simulink model "SKKP"  (R2014b)
settings: Solver=ode113  StartTime=0.0  StopTime=400  FixedStep=0.1  RelTol=1e-1  AbsTol=1e-1
undefined symbols (not defined in the file or in its folder): deg, eps_max, eps_min, H3dm, H4dm, Jdm, L, M3dm, M4dm, Newton, P, R0, rad, Raphson, s, Td, Tpp, V0, y_out
libraries: aerolibconvert2 x26, aerolibtransform2 x19, aerolibutil x7, aerolibobsolete x6, dspinverses x5, vrlib x1, aerolib6dof2 x1
(part 2 of 2)

== system SKKP/Фильтр калмана w  ==
  wizm : Inport
  wtek : Inport  Port=2
  Angular Velocity Conversion1 : aerolibconvert2/Angular Velocity Conversion  IU=rad/s  OU=deg/s
  Demux1 : Demux  Outputs=3
  Demux2 : Demux  Outputs=3
  MATLAB Function : MATLAB Function  TreatAsAtomicUnit=on
  MATLAB Function1 : MATLAB Function  TreatAsAtomicUnit=on
  MATLAB Function2 : MATLAB Function  TreatAsAtomicUnit=on
  Mux : Mux  Inputs=3
  wfilt : Outport
  wires:
  Demux1/1 -> MATLAB Function/2(meas)
  MATLAB Function1/2(yhatOut) -> Mux/2
  MATLAB Function/2(yhatOut) -> Mux/1
  MATLAB Function2/2(yhatOut) -> Mux/3
  Demux2/3 -> MATLAB Function2/1(u)
  Demux2/2 -> MATLAB Function1/1(u)
  Demux1/2 -> MATLAB Function1/2(meas)
  Demux2/1 -> MATLAB Function/1(u)
  Mux/1 -> Angular Velocity Conversion1/1
  wtek/1 -> Demux2/1
  Demux1/3 -> MATLAB Function2/2(meas)
  wizm/1 -> Demux1/1
  Angular Velocity Conversion1/1 -> wfilt/1

== system SKKP/АД/Перевод из углов в кватернионы1 ==
  fi : Inport
  Angle Conversion1 : aerolibconvert2/Angle Conversion  IU=deg  OU=rad
  Rotation Angles to Quaternions1 : aerolibtransform2/Rotation Angles to Quaternions  rotationOrder=ZYX
  Selector1 : Selector  InputPortWidth=3  Indices=[3 2 1]
  q : Outport
  wires:
  Angle Conversion1/1 -> Rotation Angles to Quaternions1/1
  Selector1/1 -> Angle Conversion1/1
  Rotation Angles to Quaternions1/1 -> q/1
  fi/1 -> Selector1/1

== system SKKP/ГИВУС/Subsystem ==
  ЧЭ1 : Inport
  ЧЭ2 : Inport  Port=2
  ЧЭ3 : Inport  Port=3
  ЧЭ4 : Inport  Port=4
  Gain4 : Gain
  wпск : Outport
  wires:
  Gain4/1 -> wпск/1
  ЧЭ1/1 -> Gain4/1

== system SKKP/Задание моментов инерции/Разворот 1 ==
  j : Inport
  Action Port : ActionPort  ActionType=then
  "j  " : Outport
  wires:
  j/1 -> "j  "/1

== system SKKP/Задание моментов инерции/Разворот 10 ==
  "j " : Inport
  Action Port : ActionPort  ActionType=then
  "j  " : Outport
  wires:
  "j "/1 -> "j  "/1

== system SKKP/Задание моментов инерции/Разворот 2 ==
  j : Inport
  Action Port : ActionPort  ActionType=then
  "j  " : Outport
  wires:
  j/1 -> "j  "/1

== system SKKP/Задание моментов инерции/Разворот 3 ==
  j : Inport
  Action Port : ActionPort  ActionType=then
  "j  " : Outport
  wires:
  j/1 -> "j  "/1

== system SKKP/Задание моментов инерции/Разворот 4 ==
  "j " : Inport
  Action Port : ActionPort  ActionType=then
  "j  " : Outport
  wires:
  "j "/1 -> "j  "/1

== system SKKP/Задание моментов инерции/Разворот 5 ==
  "j " : Inport
  Action Port : ActionPort  ActionType=then
  "j  " : Outport
  wires:
  "j "/1 -> "j  "/1

== system SKKP/Задание моментов инерции/Разворот 6 ==
  "j " : Inport
  Action Port : ActionPort  ActionType=then
  "j  " : Outport
  wires:
  "j "/1 -> "j  "/1

== system SKKP/Задание моментов инерции/Разворот 7 ==
  "j " : Inport
  Action Port : ActionPort  ActionType=then
  "j  " : Outport
  wires:
  "j "/1 -> "j  "/1

== system SKKP/Задание моментов инерции/Разворот 8 ==
  "j " : Inport
  Action Port : ActionPort  ActionType=then
  "j  " : Outport
  wires:
  "j "/1 -> "j  "/1

== system SKKP/Задание моментов инерции/Разворот 9 ==
  "j " : Inport
  Action Port : ActionPort  ActionType=then
  "j  " : Outport
  wires:
  "j "/1 -> "j  "/1

== system SKKP/КУДМ/DM5 ==
  sig1 : Inport
  1/m : Gain  Gain=1/0.0010464
  Add2 : Sum  Inputs=-+--
  Add3 : Sum
  Constant1 : Constant
  Divide1 : Product  Inputs=**
  Fcn2 : Fcn  Expr=cos(48*u[1])/17.5-cos(96*u[1])/71.5
  Gain1 : Gain  Gain=0.00095
  Gain3 : Gain  Gain=1/Jdm
  Integrator2 : Integrator
  Integrator3 : Integrator
  Kd : Gain  Gain=0.0327
  Signw : Signum  ZeroCross=off
  Transfer Fcn1 : TransferFcn  Numerator=[0.032]  Denominator=[0.3 1]
  e : Gain  Gain=1.65e-7
  h : Gain  Gain=16e-6
  w^(1/2) : Fcn  Expr=abs(u[1])^1.5
  M1 : Outport
  w1 : Outport  Port=2
  wires:
  1/m/1 -> Transfer Fcn1/1  "n"
  Transfer Fcn1/1 -> Kd/1  "i"
  Kd/1 -> Divide1/1  "Kd*i"
  Add2/1 -> M1/1, Gain3/1  "M"
  h/1 -> Add2/3  "h*w"
  Gain1/1 -> Add2/1  "Mct"
  Gain3/1 -> Integrator2/1
  Integrator2/1 -> h/1, w^(1/2)/1, w1/1, Integrator3/1, Signw/1  "W"
  Signw/1 -> Gain1/1
  Integrator3/1 -> Fcn2/1  "f"
  Fcn2/1 -> Add3/2
  Divide1/1 -> Add2/2
  e/1 -> Add2/4  "e*w^(1/2)"
  w^(1/2)/1 -> e/1
  Constant1/1 -> Add3/1
  Add3/1 -> Divide1/2
  sig1/1 -> 1/m/1

== system SKKP/КУДМ/DM6 ==
  sig2 : Inport
  1/m : Gain  Gain=1/0.0010464
  Add2 : Sum  Inputs=-+--
  Add3 : Sum
  Constant1 : Constant
  Divide1 : Product  Inputs=**
  Fcn2 : Fcn  Expr=cos(48*u[1])/17.5-cos(96*u[1])/71.5
  Gain1 : Gain  Gain=0.00095
  Gain3 : Gain  Gain=1/Jdm
  Integrator2 : Integrator
  Integrator3 : Integrator
  Kd : Gain  Gain=0.0327
  Signw : Signum  ZeroCross=off
  Transfer Fcn1 : TransferFcn  Numerator=[0.032]  Denominator=[0.3 1]
  e : Gain  Gain=1.65e-7
  h : Gain  Gain=16e-6
  w^(1/2) : Fcn  Expr=abs(u[1])^1.5
  M2 : Outport
  w2 : Outport  Port=2
  wires:
  1/m/1 -> Transfer Fcn1/1  "n"
  Transfer Fcn1/1 -> Kd/1  "i"
  Kd/1 -> Divide1/1  "Kd*i"
  Add2/1 -> M2/1, Gain3/1  "M"
  h/1 -> Add2/3  "h*w"
  Gain1/1 -> Add2/1  "Mct"
  Gain3/1 -> Integrator2/1
  Integrator2/1 -> h/1, w^(1/2)/1, w2/1, Integrator3/1, Signw/1  "W"
  Signw/1 -> Gain1/1
  Integrator3/1 -> Fcn2/1  "f"
  Fcn2/1 -> Add3/2
  Divide1/1 -> Add2/2
  e/1 -> Add2/4  "e*w^(1/2)"
  w^(1/2)/1 -> e/1
  Constant1/1 -> Add3/1
  Add3/1 -> Divide1/2
  sig2/1 -> 1/m/1

== system SKKP/КУДМ/DM7 ==
  sig3 : Inport
  1/m : Gain  Gain=1/0.0010464
  Add2 : Sum  Inputs=-+--
  Add3 : Sum
  Constant1 : Constant
  Divide1 : Product  Inputs=**
  Fcn2 : Fcn  Expr=cos(48*u[1])/17.5-cos(96*u[1])/71.5
  Gain1 : Gain  Gain=0.00095
  Gain3 : Gain  Gain=1/Jdm
  Integrator2 : Integrator
  Integrator3 : Integrator
  Kd : Gain  Gain=0.0327
  Signw : Signum  ZeroCross=off
  Transfer Fcn1 : TransferFcn  Numerator=[0.032]  Denominator=[0.3 1]
  e : Gain  Gain=1.65e-7
  h : Gain  Gain=16e-6
  w^(1/2) : Fcn  Expr=abs(u[1])^1.5
  M3 : Outport
  w3 : Outport  Port=2
  wires:
  1/m/1 -> Transfer Fcn1/1  "n"
  Transfer Fcn1/1 -> Kd/1  "i"
  Kd/1 -> Divide1/1  "Kd*i"
  Add2/1 -> M3/1, Gain3/1  "M"
  h/1 -> Add2/3  "h*w"
  Gain1/1 -> Add2/1  "Mct"
  Gain3/1 -> Integrator2/1
  Integrator2/1 -> h/1, w^(1/2)/1, w3/1, Integrator3/1, Signw/1  "W"
  Signw/1 -> Gain1/1
  Integrator3/1 -> Fcn2/1  "f"
  Fcn2/1 -> Add3/2
  Divide1/1 -> Add2/2
  e/1 -> Add2/4  "e*w^(1/2)"
  w^(1/2)/1 -> e/1
  Constant1/1 -> Add3/1
  Add3/1 -> Divide1/2
  sig3/1 -> 1/m/1

== system SKKP/КУДМ/DM8 ==
  sig4 : Inport
  1/m : Gain  Gain=1/0.0010464
  Add2 : Sum  Inputs=-+--
  Add3 : Sum
  Constant1 : Constant
  Divide1 : Product  Inputs=**
  Fcn2 : Fcn  Expr=cos(48*u[1])/17.5-cos(96*u[1])/71.5
  Gain1 : Gain  Gain=0.00095
  Gain3 : Gain  Gain=1/Jdm
  Integrator2 : Integrator
  Integrator3 : Integrator
  Kd : Gain  Gain=0.0327
  Signw : Signum  ZeroCross=off
  Transfer Fcn1 : TransferFcn  Numerator=[0.032]  Denominator=[0.3 1]
  e : Gain  Gain=1.65e-7
  h : Gain  Gain=16e-6
  w^(1/2) : Fcn  Expr=abs(u[1])^1.5
  M4 : Outport
  w4 : Outport  Port=2
  wires:
  1/m/1 -> Transfer Fcn1/1  "n"
  Transfer Fcn1/1 -> Kd/1  "i"
  Kd/1 -> Divide1/1  "Kd*i"
  Add2/1 -> Gain3/1, M4/1  "M"
  h/1 -> Add2/3  "h*w"
  Gain1/1 -> Add2/1  "Mct"
  Gain3/1 -> Integrator2/1
  Integrator2/1 -> h/1, w^(1/2)/1, w4/1, Integrator3/1, Signw/1  "W"
  Signw/1 -> Gain1/1
  Integrator3/1 -> Fcn2/1  "f"
  Fcn2/1 -> Add3/2
  Divide1/1 -> Add2/2
  e/1 -> Add2/4  "e*w^(1/2)"
  w^(1/2)/1 -> e/1
  Constant1/1 -> Add3/1
  Add3/1 -> Divide1/2
  sig4/1 -> 1/m/1

== system SKKP/КУДМ/Subsystem ==
  In1 : Inport
  Demux : Demux  Outputs=3
  If Action Subsystem1 : Subsystem  TreatAsAtomicUnit=on
  If Action Subsystem2 : Subsystem  TreatAsAtomicUnit=on
  If Action Subsystem3 : Subsystem  TreatAsAtomicUnit=on
  If Action Subsystem4 : Subsystem  TreatAsAtomicUnit=on
  If Action Subsystem5 : Subsystem  TreatAsAtomicUnit=on
  If Action Subsystem6 : Subsystem  TreatAsAtomicUnit=on
  If1 : If  IfExpression=(u1 > 1) | (u1 < -1)
  If2 : If  IfExpression=(u1 > 1) | (u1 < -1)
  If3 : If  IfExpression=(u1 > 1) | (u1 < -1)
  Merge1 : Merge
  Merge2 : Merge
  Merge3 : Merge
  Mux : Mux  Inputs=3
  Out1 : Outport
  wires:
  If1/1 -> If Action Subsystem1/Action
  Demux/1 -> If Action Subsystem1/1(in), If1/1
  If Action Subsystem1/1(B11) -> Merge3/2
  Mux/1 -> Out1/1
  In1/1 -> Demux/1
  If1/2 -> If Action Subsystem4/Action
  If Action Subsystem4/1(B11) -> Merge3/1
  Merge3/1 -> Mux/1
  If2/1 -> If Action Subsystem2/Action
  Demux/2 -> If2/1, If Action Subsystem2/1(in)
  If Action Subsystem2/1(B11) -> Merge1/2
  If2/2 -> If Action Subsystem3/Action
  If Action Subsystem3/1(B11) -> Merge1/1
  If3/1 -> If Action Subsystem5/Action
  Demux/3 -> If Action Subsystem5/1(in), If3/1
  If Action Subsystem5/1(B11) -> Merge2/2
  If3/2 -> If Action Subsystem6/Action
  If Action Subsystem6/1(B11) -> Merge2/1
  Merge2/1 -> Mux/3
  Merge1/1 -> Mux/2

== system SKKP/Момент пиропатронов/Разворот 1 ==
  M : Inport
  Action Port : ActionPort  ActionType=then
  "M " : Outport
  wires:
  M/1 -> "M "/1

== system SKKP/Момент пиропатронов/Разворот 10 ==
  M : Inport
  Action Port : ActionPort  ActionType=then
  "M " : Outport
  wires:
  M/1 -> "M "/1

== system SKKP/Момент пиропатронов/Разворот 2 ==
  M : Inport
  Action Port : ActionPort  ActionType=then
  "M " : Outport
  wires:
  M/1 -> "M "/1

== system SKKP/Момент пиропатронов/Разворот 3 ==
  M : Inport
  Action Port : ActionPort  ActionType=then
  "M " : Outport
  wires:
  M/1 -> "M "/1

== system SKKP/Момент пиропатронов/Разворот 4 ==
  M : Inport
  Action Port : ActionPort  ActionType=then
  "M " : Outport
  wires:
  M/1 -> "M "/1

== system SKKP/Момент пиропатронов/Разворот 5 ==
  M : Inport
  Action Port : ActionPort  ActionType=then
  "M " : Outport
  wires:
  M/1 -> "M "/1

== system SKKP/Момент пиропатронов/Разворот 6 ==
  M : Inport
  Action Port : ActionPort  ActionType=then
  "M " : Outport
  wires:
  M/1 -> "M "/1

== system SKKP/Момент пиропатронов/Разворот 7 ==
  M : Inport
  Action Port : ActionPort  ActionType=then
  "M " : Outport
  wires:
  M/1 -> "M "/1

== system SKKP/Момент пиропатронов/Разворот 8 ==
  M : Inport
  Action Port : ActionPort  ActionType=then
  "M " : Outport
  wires:
  M/1 -> "M "/1

== system SKKP/Момент пиропатронов/Разворот 9 ==
  M : Inport
  Action Port : ActionPort  ActionType=then
  "M " : Outport
  wires:
  M/1 -> "M "/1

== system SKKP/Объект/Quaternion Normalize  ==
  q : Inport
  Demux : Demux
  Demux1 : Demux
  Mux : Mux
  Product{,1..3} (4 alike) : Product  Inputs=*/
  Product{4,6..8} (4 alike) : Product
  Sum : Sum  Inputs=4
  sqrt : Sqrt  AlgorithmType=Newton-Raphson  SaturateOnIntegerOverflow=on
  norma(q) : Outport
  wires:
  q/1 -> Demux/1, Demux1/1
  Mux/1 -> norma(q)/1
  Product7/1 -> Sum/3
  Product4/1 -> Sum/1
  Demux1/1 -> Product4/2, Product4/1
  sqrt/1 -> Product1/2, Product/2, Product2/2, Product3/2
  Demux/4 -> Product3/1
  Demux1/3 -> Product7/2, Product7/1
  Sum/1 -> sqrt/1
  Demux/2 -> Product1/1
  Product/1 -> Mux/1
  Product6/1 -> Sum/2
  Demux/3 -> Product2/1
  Demux1/2 -> Product6/2, Product6/1
  Demux1/4 -> Product8/2, Product8/1
  Product2/1 -> Mux/3
  Product1/1 -> Mux/2
  Product3/1 -> Mux/4
  Product8/1 -> Sum/4
  Demux/1 -> Product/1

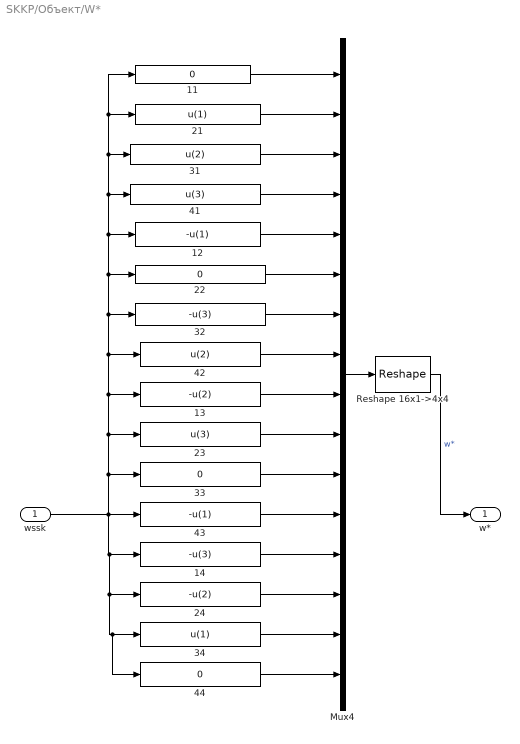
== system SKKP/Объект/W* ==
  wssk : Inport
  {11,22,33,44} (4 alike) : Fcn  Expr=0
  12 : Fcn  Expr=-u(1)
  13 : Fcn  Expr=-u(2)
  14 : Fcn  Expr=-u(3)
  21 : Fcn  Expr=u(1)
  23 : Fcn  Expr=u(3)
  24 : Fcn  Expr=-u(2)
  31 : Fcn  Expr=u(2)
  32 : Fcn  Expr=-u(3)
  34 : Fcn  Expr=u(1)
  "41 " : Fcn  Expr=u(3)
  42 : Fcn  Expr=u(2)
  43 : Fcn  Expr=-u(1)
  Mux4 : Mux  Inputs=16
  Reshape 16x1->4x4 : Reshape  OutputDimensionality=Customize  OutputDimensions=[4,4]
  w* : Outport
  wires:
  wssk/1 -> 43/1, 33/1, 23/1, 13/1, 42/1, 32/1, 22/1, 12/1, "41 "/1, 31/1, 21/1, 11/1, 14/1, 24/1, 34/1, 44/1
  31/1 -> Mux4/3
  24/1 -> Mux4/14
  33/1 -> Mux4/11
  14/1 -> Mux4/13
  13/1 -> Mux4/9
  Mux4/1 -> Reshape 16x1->4x4/1
  42/1 -> Mux4/8
  22/1 -> Mux4/6
  32/1 -> Mux4/7
  34/1 -> Mux4/15
  12/1 -> Mux4/5
  23/1 -> Mux4/10
  43/1 -> Mux4/12
  "41 "/1 -> Mux4/4
  11/1 -> Mux4/1
  21/1 -> Mux4/2
  44/1 -> Mux4/16
  Reshape 16x1->4x4/1 -> w*/1  "w*"

== system SKKP/Полетное задание/Subsystem7 ==
  q : Inport
  Angle Conversion1 : aerolibconvert2/Angle Conversion  IU=rad  OU=deg
  Direction Cosine Matrix to Euler Angles1 : aerolibobsolete/Direction Cosine Matrix to Euler Angles
  Quaternions to Direction Cosine Matrix3 : aerolibtransform2/Quaternions to  Direction Cosine Matrix
  deg : Outport
  wires:
  Quaternions to Direction Cosine Matrix3/1 -> Direction Cosine Matrix to Euler Angles1/1
  Direction Cosine Matrix to Euler Angles1/1 -> Angle Conversion1/1
  Angle Conversion1/1 -> deg/1
  q/1 -> Quaternions to Direction Cosine Matrix3/1

== system SKKP/Полетное задание/Перевод из углов в кватернионы ==
  fi : Inport
  Angle Conversion1 : aerolibconvert2/Angle Conversion  IU=deg  OU=rad
  Rotation Angles to Quaternions1 : aerolibtransform2/Rotation Angles to Quaternions  rotationOrder=ZYX
  Selector1 : Selector  InputPortWidth=3  Indices=[3 2 1]
  q : Outport
  wires:
  Angle Conversion1/1 -> Rotation Angles to Quaternions1/1
  Selector1/1 -> Angle Conversion1/1
  Rotation Angles to Quaternions1/1 -> q/1
  fi/1 -> Selector1/1

== system SKKP/Полетное задание/Перевод из углов в кватернионы  ==
  fi : Inport
  Angle Conversion1 : aerolibconvert2/Angle Conversion  IU=deg  OU=rad
  Rotation Angles to Quaternions1 : aerolibtransform2/Rotation Angles to Quaternions  rotationOrder=ZYX
  Selector1 : Selector  InputPortWidth=3  Indices=[3 2 1]
  q : Outport
  wires:
  Angle Conversion1/1 -> Rotation Angles to Quaternions1/1
  Selector1/1 -> Angle Conversion1/1
  Rotation Angles to Quaternions1/1 -> q/1
  fi/1 -> Selector1/1

== system SKKP/Полетное задание/Признак  разворота ==
  Action Port : ActionPort  ActionType=then
  Constant : Constant
  priz_raz : Outport
  wires:
  Constant/1 -> priz_raz/1

== system SKKP/Полетное задание/Признак  разворота1 ==
  Action Port : ActionPort  ActionType=else
  Constant : Constant  Value=0
  priz_raz : Outport
  wires:
  Constant/1 -> priz_raz/1

== system SKKP/Полетное задание/Разворот 1 ==
  fi_zad1 : Inport
  fi01 : Inport  Port=2
  Action Port : ActionPort  ActionType=then
  "fi_zad1  " : Outport
  "fi01  " : Outport  Port=2
  wires:
  fi01/1 -> "fi01  "/1
  fi_zad1/1 -> "fi_zad1  "/1

== system SKKP/Полетное задание/Разворот 10 ==
  fi_zad1 : Inport
  fi01 : Inport  Port=2
  Action Port : ActionPort  ActionType=then
  "fi_zad1  " : Outport
  "fi01  " : Outport  Port=2
  wires:
  fi_zad1/1 -> "fi_zad1  "/1
  fi01/1 -> "fi01  "/1

== system SKKP/Полетное задание/Разворот 2 ==
  fi_zad1 : Inport
  fi01 : Inport  Port=2
  Action Port : ActionPort  ActionType=then
  "fi_zad1  " : Outport
  "fi01  " : Outport  Port=2
  wires:
  fi_zad1/1 -> "fi_zad1  "/1
  fi01/1 -> "fi01  "/1

== system SKKP/Полетное задание/Разворот 3 ==
  fi_zad1 : Inport
  fi01 : Inport  Port=2
  Action Port : ActionPort  ActionType=then
  "fi_zad1  " : Outport
  "fi01  " : Outport  Port=2
  wires:
  fi01/1 -> "fi01  "/1
  fi_zad1/1 -> "fi_zad1  "/1

== system SKKP/Полетное задание/Разворот 4 ==
  fi_zad1 : Inport
  fi01 : Inport  Port=2
  Action Port : ActionPort  ActionType=then
  "fi_zad1  " : Outport
  "fi01  " : Outport  Port=2
  wires:
  fi_zad1/1 -> "fi_zad1  "/1
  fi01/1 -> "fi01  "/1

== system SKKP/Полетное задание/Разворот 5 ==
  fi_zad1 : Inport
  fi01 : Inport  Port=2
  Action Port : ActionPort  ActionType=then
  "fi_zad1  " : Outport
  "fi01  " : Outport  Port=2
  wires:
  fi01/1 -> "fi01  "/1
  fi_zad1/1 -> "fi_zad1  "/1

== system SKKP/Полетное задание/Разворот 6 ==
  fi_zad1 : Inport
  fi01 : Inport  Port=2
  Action Port : ActionPort  ActionType=then
  "fi_zad1  " : Outport
  "fi01  " : Outport  Port=2
  wires:
  fi_zad1/1 -> "fi_zad1  "/1
  fi01/1 -> "fi01  "/1

== system SKKP/Полетное задание/Разворот 7 ==
  fi_zad1 : Inport
  fi01 : Inport  Port=2
  Action Port : ActionPort  ActionType=then
  "fi_zad1  " : Outport
  "fi01  " : Outport  Port=2
  wires:
  fi01/1 -> "fi01  "/1
  fi_zad1/1 -> "fi_zad1  "/1

== system SKKP/Полетное задание/Разворот 8 ==
  fi_zad1 : Inport
  fi01 : Inport  Port=2
  Action Port : ActionPort  ActionType=then
  "fi_zad1  " : Outport
  "fi01  " : Outport  Port=2
  wires:
  fi_zad1/1 -> "fi_zad1  "/1
  fi01/1 -> "fi01  "/1

== system SKKP/Полетное задание/Разворот 9 ==
  fi_zad1 : Inport
  fi01 : Inport  Port=2
  Action Port : ActionPort  ActionType=then
  "fi_zad1  " : Outport
  "fi01  " : Outport  Port=2
  wires:
  fi01/1 -> "fi01  "/1
  fi_zad1/1 -> "fi_zad1  "/1

== system SKKP/Програмный разворот /Subsystem5 ==
  qvat : Inport
  Mux2 : Mux  Inputs=3
  q0 : Fcn  Expr=acos(u(1))*2/pi*180
  q1 : Fcn  Expr=u(2)/(sqrt(u(2)^2+u(3)^2+u(4)^2))
  q2 : Fcn  Expr=u(3)/(sqrt(u(2)^2+u(3)^2+u(4)^2))
  q3 : Fcn  Expr=u(4)/(sqrt(u(2)^2+u(3)^2+u(4)^2))
  e : Outport  InitialOutput=0
  fi : Outport  Port=2  InitialOutput=0
  wires:
  Mux2/1 -> e/1
  q2/1 -> Mux2/2
  q3/1 -> Mux2/3
  q0/1 -> fi/1
  qvat/1 -> q0/1, q1/1, q2/1, q3/1
  q1/1 -> Mux2/1

== system SKKP/Програмный разворот /angle2qvat3 ==
  fi : Inport
  e : Inport  Port=2
  1/2 : Gain  Gain=0.5/180*pi  SaturateOnIntegerOverflow=on  OutDataTypeStr=Inherit: Same as input  ParamDataTypeStr=Inherit: Same as input
  Display : Display
  Mux1 : Mux  Inputs=3
  Mux2 : Mux
  q0 : Fcn  Expr=u(2)
  q1 : Fcn  Expr=u(1)*u(3)
  q2 : Fcn  Expr=u(1)*u(4)
  q3 : Fcn  Expr=u(1)*u(5)
  sincos : Trigonometry  Operator=sincos
  Quat : Outport  InitialOutput=0
  wires:
  e/1 -> Mux1/3
  q1/1 -> Mux2/2
  1/2/1 -> sincos/1
  sincos/2 -> Mux1/2
  Mux1/1 -> q3/1, q2/1, q1/1, q0/1
  fi/1 -> 1/2/1
  q0/1 -> Mux2/1
  q3/1 -> Mux2/4
  q2/1 -> Mux2/3
  Mux2/1 -> Quat/1, Display/1
  sincos/1 -> Mux1/1

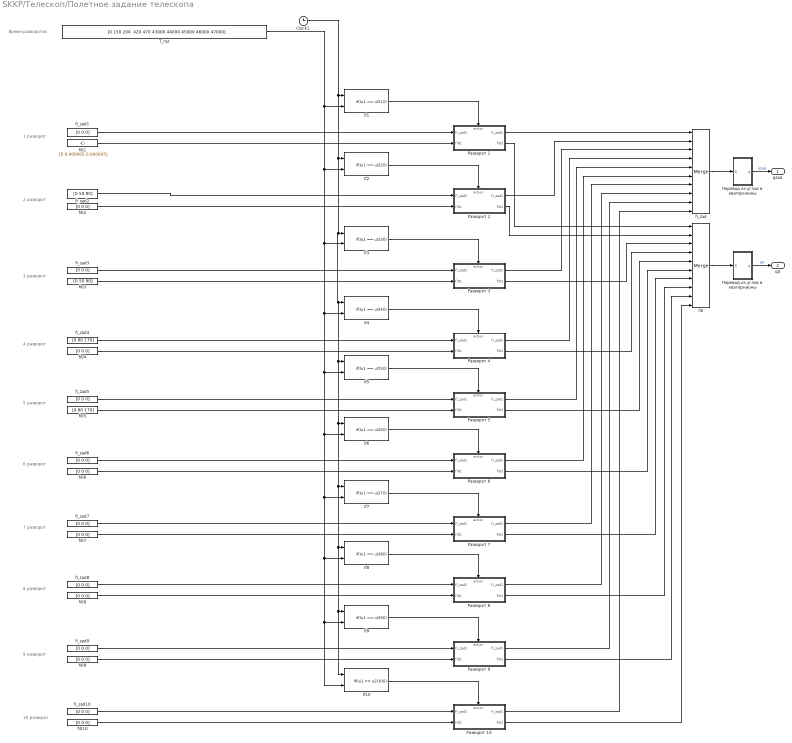
== system SKKP/Телескоп/Полетное задание телескопа ==
  note: 1 разворот
  note: 2 разворот
  note: 3 разворот
  note: 4 разворот
  note: 5 разворот
  note: 6 разворот
  note: 7 разворот
  note: 8 разворот
  note: 9 разворот
  note: 10 разворот
  note: Время разворотов
  Clock1 : Clock
  If1 : If  NumInputs=2  IfExpression=(u1 == u2(1))  ShowElse=off
  If10 : If  NumInputs=2  IfExpression=(u1 == u2(10))  ShowElse=off
  If2 : If  NumInputs=2  IfExpression=(u1 == u2(2))  ShowElse=off
  If3 : If  NumInputs=2  IfExpression=(u1 == u2(3))  ShowElse=off
  If4 : If  NumInputs=2  IfExpression=(u1 == u2(4))  ShowElse=off
  If5 : If  NumInputs=2  IfExpression=(u1 == u2(5))  ShowElse=off
  If6 : If  NumInputs=2  IfExpression=(u1 == u2(6))  ShowElse=off
  If7 : If  NumInputs=2  IfExpression=(u1 == u2(7))  ShowElse=off
  If8 : If  NumInputs=2  IfExpression=(u1 == u2(8))  ShowElse=off
  If9 : If  NumInputs=2  IfExpression=(u1 == u2(9))  ShowElse=off
  T_raz : Constant  Value="[0 150 200  420 470 43000 44000 45000 46000 47000]"
  fi0 : Merge  Inputs=10
  fi01 : Constant  Value=[0 0.000005 0.000005]
  fi010 : Constant  Value=[0 0 0]
  fi02 : Constant  Value=[0 0 0]
  fi03 : Constant  Value=[0 50 90]
  fi04 : Constant  Value=[0 0 0]
  fi05 : Constant  Value=[0 80 170]
  fi06 : Constant  Value=[0 0 0]
  fi07 : Constant  Value=[0 0 0]
  fi08 : Constant  Value=[0 0 0]
  fi09 : Constant  Value=[0 0 0]
  fi_zad : Merge  Inputs=10
  fi_zad{1,3,5..10} (8 alike) : Constant  Value=[0 0 0]
  fi_zad2 : Constant  Value=[0 50 90]
  fi_zad4 : Constant  Value=[0 80 170]
  Перевод из углов в кватернионы : Subsystem
  "Перевод из углов в кватернионы " : Subsystem
  Разворот 1 : Subsystem  TreatAsAtomicUnit=on
  Разворот 10 : Subsystem  TreatAsAtomicUnit=on
  Разворот 2 : Subsystem  TreatAsAtomicUnit=on
  Разворот 3 : Subsystem  TreatAsAtomicUnit=on
  Разворот 4 : Subsystem  TreatAsAtomicUnit=on
  Разворот 5 : Subsystem  TreatAsAtomicUnit=on
  Разворот 6 : Subsystem  TreatAsAtomicUnit=on
  Разворот 7 : Subsystem  TreatAsAtomicUnit=on
  Разворот 8 : Subsystem  TreatAsAtomicUnit=on
  Разворот 9 : Subsystem  TreatAsAtomicUnit=on
  qzad : Outport
  q0 : Outport  Port=2
  wires:
  fi01/1 -> Разворот 1/2(fi01)
  fi_zad1/1 -> Разворот 1/1(fi_zad1)
  If1/1 -> Разворот 1/Action
  fi02/1 -> Разворот 2/2(fi01)
  fi_zad2/1 -> Разворот 2/1(fi_zad1)
  If2/1 -> Разворот 2/Action
  fi03/1 -> Разворот 3/2(fi01)
  fi_zad3/1 -> Разворот 3/1(fi_zad1)
  If3/1 -> Разворот 3/Action
  fi04/1 -> Разворот 4/2(fi01)
  fi_zad4/1 -> Разворот 4/1(fi_zad1)
  If4/1 -> Разворот 4/Action
  fi05/1 -> Разворот 5/2(fi01)
  fi_zad5/1 -> Разворот 5/1(fi_zad1)
  If5/1 -> Разворот 5/Action
  fi06/1 -> Разворот 6/2(fi01)
  fi_zad6/1 -> Разворот 6/1(fi_zad1)
  If6/1 -> Разворот 6/Action
  fi07/1 -> Разворот 7/2(fi01)
  fi_zad7/1 -> Разворот 7/1(fi_zad1)
  If7/1 -> Разворот 7/Action
  fi08/1 -> Разворот 8/2(fi01)
  fi_zad8/1 -> Разворот 8/1(fi_zad1)
  If8/1 -> Разворот 8/Action
  fi09/1 -> Разворот 9/2(fi01)
  fi_zad9/1 -> Разворот 9/1(fi_zad1)
  If9/1 -> Разворот 9/Action
  fi010/1 -> Разворот 10/2(fi01)
  fi_zad10/1 -> Разворот 10/1(fi_zad1)
  If10/1 -> Разворот 10/Action
  Разворот 1/1("fi_zad1  ") -> fi_zad/1
  Разворот 1/2("fi01  ") -> fi0/1
  Разворот 2/1("fi_zad1  ") -> fi_zad/2
  Разворот 3/1("fi_zad1  ") -> fi_zad/3
  Разворот 4/1("fi_zad1  ") -> fi_zad/4
  Разворот 5/1("fi_zad1  ") -> fi_zad/5
  Разворот 6/1("fi_zad1  ") -> fi_zad/6
  Разворот 7/1("fi_zad1  ") -> fi_zad/7
  Разворот 8/1("fi_zad1  ") -> fi_zad/8
  Разворот 9/1("fi_zad1  ") -> fi_zad/9
  Разворот 10/1("fi_zad1  ") -> fi_zad/10
  Разворот 2/2("fi01  ") -> fi0/2
  Разворот 3/2("fi01  ") -> fi0/3
  Разворот 4/2("fi01  ") -> fi0/4
  Разворот 5/2("fi01  ") -> fi0/5
  Разворот 6/2("fi01  ") -> fi0/6
  Разворот 7/2("fi01  ") -> fi0/7
  Разворот 8/2("fi01  ") -> fi0/8
  Разворот 9/2("fi01  ") -> fi0/9
  Разворот 10/2("fi01  ") -> fi0/10
  Перевод из углов в кватернионы/1(q) -> qzad/1  "qzad"
  "Перевод из углов в кватернионы "/1(q) -> q0/1  "q0"
  T_raz/1 -> If2/2, If4/2, If6/2, If10/2, If9/2, If8/2, If7/2, If5/2, If3/2, If1/2
  Clock1/1 -> If10/1, If9/1, If8/1, If7/1, If6/1, If5/1, If4/1, If3/1, If2/1, If1/1
  fi_zad/1 -> Перевод из углов в кватернионы/1(fi)
  fi0/1 -> "Перевод из углов в кватернионы "/1(fi)

== system SKKP/КУДМ/Subsystem/If Action Subsystem1 ==
  in : Inport
  Action Port : ActionPort  ActionType=then
  B11 : Outport
  wires:
  in/1 -> B11/1

== system SKKP/КУДМ/Subsystem/If Action Subsystem2 ==
  in : Inport
  Action Port : ActionPort  ActionType=then
  B11 : Outport
  wires:
  in/1 -> B11/1

== system SKKP/КУДМ/Subsystem/If Action Subsystem3 ==
  Action Port : ActionPort  ActionType=else
  Constant : Constant  Value=0
  B11 : Outport
  wires:
  Constant/1 -> B11/1

== system SKKP/КУДМ/Subsystem/If Action Subsystem4 ==
  Action Port : ActionPort  ActionType=else
  Constant : Constant  Value=0
  B11 : Outport
  wires:
  Constant/1 -> B11/1

== system SKKP/КУДМ/Subsystem/If Action Subsystem5 ==
  in : Inport
  Action Port : ActionPort  ActionType=then
  B11 : Outport
  wires:
  in/1 -> B11/1

== system SKKP/КУДМ/Subsystem/If Action Subsystem6 ==
  Action Port : ActionPort  ActionType=else
  Constant : Constant  Value=0
  B11 : Outport
  wires:
  Constant/1 -> B11/1

== system SKKP/Телескоп/Полетное задание телескопа/Перевод из углов в кватернионы ==
  fi : Inport
  Angle Conversion1 : aerolibconvert2/Angle Conversion  IU=deg  OU=rad
  Rotation Angles to Quaternions1 : aerolibtransform2/Rotation Angles to Quaternions  rotationOrder=ZYX
  Selector1 : Selector  InputPortWidth=3  Indices=[3 2 1]
  q : Outport
  wires:
  fi/1 -> Selector1/1
  Rotation Angles to Quaternions1/1 -> q/1
  Selector1/1 -> Angle Conversion1/1
  Angle Conversion1/1 -> Rotation Angles to Quaternions1/1

== system SKKP/Телескоп/Полетное задание телескопа/Перевод из углов в кватернионы  ==
  fi : Inport
  Angle Conversion1 : aerolibconvert2/Angle Conversion  IU=deg  OU=rad
  Rotation Angles to Quaternions1 : aerolibtransform2/Rotation Angles to Quaternions  rotationOrder=ZYX
  Selector1 : Selector  InputPortWidth=3  Indices=[3 2 1]
  q : Outport
  wires:
  fi/1 -> Selector1/1
  Rotation Angles to Quaternions1/1 -> q/1
  Selector1/1 -> Angle Conversion1/1
  Angle Conversion1/1 -> Rotation Angles to Quaternions1/1

== system SKKP/Телескоп/Полетное задание телескопа/Разворот 1 ==
  fi_zad1 : Inport
  fi01 : Inport  Port=2
  Action Port : ActionPort  ActionType=then
  "fi_zad1  " : Outport
  "fi01  " : Outport  Port=2
  wires:
  fi_zad1/1 -> "fi_zad1  "/1
  fi01/1 -> "fi01  "/1

== system SKKP/Телескоп/Полетное задание телескопа/Разворот 10 ==
  fi_zad1 : Inport
  fi01 : Inport  Port=2
  Action Port : ActionPort  ActionType=then
  "fi_zad1  " : Outport
  "fi01  " : Outport  Port=2
  wires:
  fi01/1 -> "fi01  "/1
  fi_zad1/1 -> "fi_zad1  "/1

== system SKKP/Телескоп/Полетное задание телескопа/Разворот 2 ==
  fi_zad1 : Inport
  fi01 : Inport  Port=2
  Action Port : ActionPort  ActionType=then
  "fi_zad1  " : Outport
  "fi01  " : Outport  Port=2
  wires:
  fi01/1 -> "fi01  "/1
  fi_zad1/1 -> "fi_zad1  "/1

== system SKKP/Телескоп/Полетное задание телескопа/Разворот 3 ==
  fi_zad1 : Inport
  fi01 : Inport  Port=2
  Action Port : ActionPort  ActionType=then
  "fi_zad1  " : Outport
  "fi01  " : Outport  Port=2
  wires:
  fi_zad1/1 -> "fi_zad1  "/1
  fi01/1 -> "fi01  "/1

== system SKKP/Телескоп/Полетное задание телескопа/Разворот 4 ==
  fi_zad1 : Inport
  fi01 : Inport  Port=2
  Action Port : ActionPort  ActionType=then
  "fi_zad1  " : Outport
  "fi01  " : Outport  Port=2
  wires:
  fi01/1 -> "fi01  "/1
  fi_zad1/1 -> "fi_zad1  "/1

== system SKKP/Телескоп/Полетное задание телескопа/Разворот 5 ==
  fi_zad1 : Inport
  fi01 : Inport  Port=2
  Action Port : ActionPort  ActionType=then
  "fi_zad1  " : Outport
  "fi01  " : Outport  Port=2
  wires:
  fi_zad1/1 -> "fi_zad1  "/1
  fi01/1 -> "fi01  "/1

== system SKKP/Телескоп/Полетное задание телескопа/Разворот 6 ==
  fi_zad1 : Inport
  fi01 : Inport  Port=2
  Action Port : ActionPort  ActionType=then
  "fi_zad1  " : Outport
  "fi01  " : Outport  Port=2
  wires:
  fi01/1 -> "fi01  "/1
  fi_zad1/1 -> "fi_zad1  "/1

== system SKKP/Телескоп/Полетное задание телескопа/Разворот 7 ==
  fi_zad1 : Inport
  fi01 : Inport  Port=2
  Action Port : ActionPort  ActionType=then
  "fi_zad1  " : Outport
  "fi01  " : Outport  Port=2
  wires:
  fi_zad1/1 -> "fi_zad1  "/1
  fi01/1 -> "fi01  "/1

== system SKKP/Телескоп/Полетное задание телескопа/Разворот 8 ==
  fi_zad1 : Inport
  fi01 : Inport  Port=2
  Action Port : ActionPort  ActionType=then
  "fi_zad1  " : Outport
  "fi01  " : Outport  Port=2
  wires:
  fi01/1 -> "fi01  "/1
  fi_zad1/1 -> "fi_zad1  "/1

== system SKKP/Телескоп/Полетное задание телескопа/Разворот 9 ==
  fi_zad1 : Inport
  fi01 : Inport  Port=2
  Action Port : ActionPort  ActionType=then
  "fi_zad1  " : Outport
  "fi01  " : Outport  Port=2
  wires:
  fi_zad1/1 -> "fi_zad1  "/1
  fi01/1 -> "fi01  "/1

== matlab function SKKP/Фильтр калмана w /MATLAB Function ==
  data: u input; xhatOut output; meas input; yhatOut output
function [xhatOut, yhatOut] = KALMAN(u,meas)
% This Embedded MATLAB Function implements a very simple Kalman filter.
%
% It implements a Kalman filter for estimating both the state and output
% of a linear, discrete-time, time-invariant, system given by the following
% state-space equations:
%
% x(k) = 0.914 x(k-1) + 0.25 u(k) + w(k)
% y(k) = 0.344 x(k-1) + v(k)
%
% where w(k) has a variance of 0.01 and v(k) has a variance of 0.1.

% Author: Phil Goddard (phil@goddardconsulting.ca)
% Date: Q2, 2011.

% Define storage for the variables that need to persist
% between time periods.
persistent P xhat A B C Q R
if isempty(P)
% First time through the code so do some initialization
   xhat = 0;
   P = 0;
   A = 0.914;
   B = 0.25;
   C = 0.344;
   Q = 0.01^2;
   R = 0.1^2;
end
% Propagate the state estimate and covariance matrix:
xhat = A*xhat + B*u;
P = A*P*A' + Q;
% Calculate the Kalman gain
K = P*C'/(C*P*C' + R);
% Calculate the measurement residual
resid = meas - C*xhat;
% Update the state and error covariance estimate
xhat = xhat + K*resid;
P = (eye(size(K,1))-K*C)*P;
% Post the results
xhatOut = xhat;
yhatOut = C*xhatOut;

== matlab function SKKP/Фильтр калмана w /MATLAB Function1 ==
  data: u input; xhatOut output; meas input; yhatOut output
function [xhatOut, yhatOut] = KALMAN(u,meas)
% This Embedded MATLAB Function implements a very simple Kalman filter.
%
% It implements a Kalman filter for estimating both the state and output
% of a linear, discrete-time, time-invariant, system given by the following
% state-space equations:
%
% x(k) = 0.914 x(k-1) + 0.25 u(k) + w(k)
% y(k) = 0.344 x(k-1) + v(k)
%
% where w(k) has a variance of 0.01 and v(k) has a variance of 0.1.

% Author: Phil Goddard (phil@goddardconsulting.ca)
% Date: Q2, 2011.

% Define storage for the variables that need to persist
% between time periods.
persistent P xhat A B C Q R
if isempty(P)
% First time through the code so do some initialization
   xhat = 0;
   P = 0;
   A = 0.914;
   B = 0.25;
   C = 0.344;
   Q = 0.01^2;
   R = 0.1^2;
end
% Propagate the state estimate and covariance matrix:
xhat = A*xhat + B*u;
P = A*P*A' + Q;
% Calculate the Kalman gain
K = P*C'/(C*P*C' + R);
% Calculate the measurement residual
resid = meas - C*xhat;
% Update the state and error covariance estimate
xhat = xhat + K*resid;
P = (eye(size(K,1))-K*C)*P;
% Post the results
xhatOut = xhat;
yhatOut = C*xhatOut;

== matlab function SKKP/Объект/MATLAB Function ==
  data: a input; xECI output; e input; i input; o input; w input; v input; vECI output
function [xECI,vECI] = kepl2eci(a,e,i,o,w,v)

% KEPL2ECI - Keplerian to ECI transformation.
% [xECI,vECI] = kepl2eci(a,e,i,o,w,v)
%
% Calculates the Nx3 position trajectory 'xECI' and Nx3 velocity 
% trajectory 'vECI' in Earth-centered-inertial coordinates given 
% Keplerian orbit element Nx1 sequences (a,e,i,o,w,v).  Scalar 
% values for any of the inputs are acceptable.  Units for 'xECI' 
% and 'vECI' are km and km/sec, respectively. 
%
% The Keplerian elements are:
%   a  :  semimajor axis (km)
%   e  :  eccentricity (unitless)
%   i  :  inclination (rad)
%   o  :  right ascension of the
%           ascending node (rad)
%   w  :  argument of perigee (rad)
%   v  :  true anomaly (rad)
%
% P.G. Bonanni
% 3/10/95


% Fix inputs
a = a(:);
e = e(:);
i = i(:);
o = o(:);
w = w(:);
v = v(:);

% Earth gravity constant
u = 398600.607;  % km^3/s^2

% Basic quantities
sini = sin(i);  cosi = cos(i);
sino = sin(o);  coso = cos(o);
sinw = sin(w);  cosw = cos(w);
Px =  coso.*cosw - sino.*sinw.*cosi;
Py =  sino.*cosw + coso.*sinw.*cosi;
Pz =  sinw.*sini;
Qx = -sino.*cosw.*cosi - coso.*sinw;
Qy =  coso.*cosw.*cosi - sino.*sinw;
Qz =  cosw.*sini;

% Eccentric anomaly
v = pvrads(v);  cosv = cos(v);
E = sign(v) .* acos((e+cosv)./(1+e.*cosv));
E = pvrad(E);

% More quantities
sinE = sin(E);
cosE = cos(E);
p  = a .* (cosE - e);
q  = a .* sqrt(1 - e.^2) .* sinE;
p1 = - sqrt(u*a)           .* sinE ./ (a .* (1 - e.*cosE));
q1 =   sqrt(u*a.*(1-e.^2)) .* cosE ./ (a .* (1 - e.*cosE));

% ECI position
xECI = [Px.*p  + Qx.*q, ...
        Py.*p  + Qy.*q, ...
        Pz.*p  + Qz.*q      ];

% ECI velocity
vECI = [Px.*p1 + Qx.*q1, ...
        Py.*p1 + Qy.*q1, ...
        Pz.*p1 + Qz.*q1      ];
    
    function angle1 = pvrad(angle)

% PVRAD - Principal value in radians.
% angle1 = pvrad(angle)
%
% This function converts angles outside the 
% range [0,2*pi] to their equivalent in that 
% range.  Both scalar and matrix inputs are 
% valid. 
%
% P.G. Bonanni
% 11/10/94

twopi = 2*pi;
angle1 = angle - floor(angle/twopi)*twopi;

function angle1 = pvrads(angle)

% PVRADS - Symmetric principal value in radians.
% angle1 = pvrads(angle)
%
% This function converts angles outside the 
% range [-pi,pi] to their equivalent in that 
% range.  Both scalar and matrix inputs are 
% valid. 
%
% P.G. Bonanni
% 11/10/94


twopi = 2*pi;
angle1 = angle - floor((angle+pi)/twopi)*twopi;

== matlab function SKKP/Фильтр калмана w /MATLAB Function2 ==
  data: u input; xhatOut output; meas input; yhatOut output
function [xhatOut, yhatOut] = KALMAN(u,meas)
% This Embedded MATLAB Function implements a very simple Kalman filter.
%
% It implements a Kalman filter for estimating both the state and output
% of a linear, discrete-time, time-invariant, system given by the following
% state-space equations:
%
% x(k) = 0.914 x(k-1) + 0.25 u(k) + w(k)
% y(k) = 0.344 x(k-1) + v(k)
%
% where w(k) has a variance of 0.01 and v(k) has a variance of 0.1.

% Author: Phil Goddard (phil@goddardconsulting.ca)
% Date: Q2, 2011.

% Define storage for the variables that need to persist
% between time periods.
persistent P xhat A B C Q R
if isempty(P)
% First time through the code so do some initialization
   xhat = 0;
   P = 0;
   A = 0.914;
   B = 0.25;
   C = 0.344;
   Q = 0.01^2;
   R = 0.1^2;
end
% Propagate the state estimate and covariance matrix:
xhat = A*xhat + B*u;
P = A*P*A' + Q;
% Calculate the Kalman gain
K = P*C'/(C*P*C' + R);
% Calculate the measurement residual
resid = meas - C*xhat;
% Update the state and error covariance estimate
xhat = xhat + K*resid;
P = (eye(size(K,1))-K*C)*P;
% Post the results
xhatOut = xhat;
yhatOut = C*xhatOut;

== matlab function SKKP/Фильтр калмана q /MATLAB Function ==
  data: u input; xhatOut output; meas input; yhatOut output
function [xhatOut, yhatOut] = KALMAN(u,meas)
% This Embedded MATLAB Function implements a very simple Kalman filter.
%
% It implements a Kalman filter for estimating both the state and output
% of a linear, discrete-time, time-invariant, system given by the following
% state-space equations:
%
% x(k) = 0.914 x(k-1) + 0.25 u(k) + w(k)
% y(k) = 0.344 x(k-1) + v(k)
%
% where w(k) has a variance of 0.01 and v(k) has a variance of 0.1.

% Author: Phil Goddard (phil@goddardconsulting.ca)
% Date: Q2, 2011.

% Define storage for the variables that need to persist
% between time periods.
persistent P xhat A B C Q R
if isempty(P)
% First time through the code so do some initialization
   xhat = 0;
   P = 0;
   A = 0.914;
   B = 0.25;
   C = 0.344;
   Q = 0.01^2;
   R = 0.1^2;
end
% Propagate the state estimate and covariance matrix:
xhat = A*xhat + B*u;
P = A*P*A' + Q;
% Calculate the Kalman gain
K = P*C'/(C*P*C' + R);
% Calculate the measurement residual
resid = meas - C*xhat;
% Update the state and error covariance estimate
xhat = xhat + K*resid;
P = (eye(size(K,1))-K*C)*P;
% Post the results
xhatOut = xhat;
yhatOut = C*xhatOut;

== matlab function SKKP/Фильтр калмана q /MATLAB Function1 ==
  data: u input; xhatOut output; meas input; yhatOut output
function [xhatOut, yhatOut] = KALMAN(u,meas)
% This Embedded MATLAB Function implements a very simple Kalman filter.
%
% It implements a Kalman filter for estimating both the state and output
% of a linear, discrete-time, time-invariant, system given by the following
% state-space equations:
%
% x(k) = 0.914 x(k-1) + 0.25 u(k) + w(k)
% y(k) = 0.344 x(k-1) + v(k)
%
% where w(k) has a variance of 0.01 and v(k) has a variance of 0.1.

% Author: Phil Goddard (phil@goddardconsulting.ca)
% Date: Q2, 2011.

% Define storage for the variables that need to persist
% between time periods.
persistent P xhat A B C Q R
if isempty(P)
% First time through the code so do some initialization
   xhat = 0;
   P = 0;
   A = 0.914;
   B = 0.25;
   C = 0.344;
   Q = 0.01^2;
   R = 0.1^2;
end
% Propagate the state estimate and covariance matrix:
xhat = A*xhat + B*u;
P = A*P*A' + Q;
% Calculate the Kalman gain
K = P*C'/(C*P*C' + R);
% Calculate the measurement residual
resid = meas - C*xhat;
% Update the state and error covariance estimate
xhat = xhat + K*resid;
P = (eye(size(K,1))-K*C)*P;
% Post the results
xhatOut = xhat;
yhatOut = C*xhatOut;

== matlab function SKKP/Фильтр калмана q /MATLAB Function2 ==
  data: u input; xhatOut output; meas input; yhatOut output
function [xhatOut, yhatOut] = KALMAN(u,meas)
% This Embedded MATLAB Function implements a very simple Kalman filter.
%
% It implements a Kalman filter for estimating both the state and output
% of a linear, discrete-time, time-invariant, system given by the following
% state-space equations:
%
% x(k) = 0.914 x(k-1) + 0.25 u(k) + w(k)
% y(k) = 0.344 x(k-1) + v(k)
%
% where w(k) has a variance of 0.01 and v(k) has a variance of 0.1.

% Author: Phil Goddard (phil@goddardconsulting.ca)
% Date: Q2, 2011.

% Define storage for the variables that need to persist
% between time periods.
persistent P xhat A B C Q R
if isempty(P)
% First time through the code so do some initialization
   xhat = 0;
   P = 0;
   A = 0.914;
   B = 0.25;
   C = 0.344;
   Q = 0.01^2;
   R = 0.1^2;
end
% Propagate the state estimate and covariance matrix:
xhat = A*xhat + B*u;
P = A*P*A' + Q;
% Calculate the Kalman gain
K = P*C'/(C*P*C' + R);
% Calculate the measurement residual
resid = meas - C*xhat;
% Update the state and error covariance estimate
xhat = xhat + K*resid;
P = (eye(size(K,1))-K*C)*P;
% Post the results
xhatOut = xhat;
yhatOut = C*xhatOut;

== matlab function SKKP/Фильтр калмана q /MATLAB Function3 ==
  data: u input; xhatOut output; meas input; yhatOut output
function [xhatOut, yhatOut] = KALMAN(u,meas)
% This Embedded MATLAB Function implements a very simple Kalman filter.
%
% It implements a Kalman filter for estimating both the state and output
% of a linear, discrete-time, time-invariant, system given by the following
% state-space equations:
%
% x(k) = 0.914 x(k-1) + 0.25 u(k) + w(k)
% y(k) = 0.344 x(k-1) + v(k)
%
% where w(k) has a variance of 0.01 and v(k) has a variance of 0.1.

% Author: Phil Goddard (phil@goddardconsulting.ca)
% Date: Q2, 2011.

% Define storage for the variables that need to persist
% between time periods.
persistent P xhat A B C Q R
if isempty(P)
% First time through the code so do some initialization
   xhat = 0;
   P = 0;
   A = 0.914;
   B = 0.25;
   C = 0.344;
   Q = 0.01^2;
   R = 0.1^2;
end
% Propagate the state estimate and covariance matrix:
xhat = A*xhat + B*u;
P = A*P*A' + Q;
% Calculate the Kalman gain
K = P*C'/(C*P*C' + R);
% Calculate the measurement residual
resid = meas - C*xhat;
% Update the state and error covariance estimate
xhat = xhat + K*resid;
P = (eye(size(K,1))-K*C)*P;
% Post the results
xhatOut = xhat;
yhatOut = C*xhatOut;

== stateflow chart SKKP/Програмный разворот /Формирование Fip Omgp ==
  settings: updateMethod=DISCRETE  sampleTime=0.1
  state init
    entry:
    p_init=0;
    t_tek=0;
    Omgp=0;
    Fip=0;
    t_r=omg_max/eps_max;
    fi_r=t_r^2*eps_max/2;
    if (fi_r<(fi/2))
    t1=t_r*10;
    t2=(fi-2*fi_r)/omg_max*10+t1;
    t3=t1+t2;
    else
    t1=sqrt(fi/eps_max)*10;
    t2=t1;
    t3=2*t1;
    end;
    traz=[t1 t2 t3]
    during:
    p_init=1;
  state init1
    entry:
    Fip=0;
    p_init=0;
    t_tek=0;
    t_r=omg_max/eps_max;
    fi_r=t_r^2*eps_max/2;
    if (fi_r<(fi/2))
    t1=t_r*10;
    t2=(fi-2*fi_r)/omg_max*10+t1;
    t3=t1+t2;
    else
    t1=sqrt(fi/eps_max)*10;
    t2=t1;
    t3=2*t1;
    end;
    traz=[t1 t2 t3]
    during:
    p_init=1;
  state all_stop
    during:
    Eps=0;
    Omgp=0;
    Fip=fi;
  state rot
    during:
    Eps=0;
    t_tek=t_tek+1;
    Omgp=omg_max;
    Fip=Fip+Omgp*0.1;
  state deccel
    during:
    Eps=-eps_max;
    t_tek=t_tek+1 ;
    Omgp=Omgp+Eps*0.1 ;
    Fip=Fip+Omgp*0.1;
  state accel
    during:
    Eps=eps_max;
    t_tek=t_tek+1;
    Omgp=Omgp+Eps*0.1;
    Fip=Fip+Omgp*0.1;
  all_stop -> init1 : [priz_raz==1]
  (default) -> init : [priz_raz==1]
  deccel -> all_stop : [t_tek>=t3-1]
  init -> accel : [p_init==1]
  init1 -> accel
  accel -> rot : [t_tek>=t1-1]
  rot -> deccel : [t_tek>=t2-1]
  data: Fip output; Omgp output; Eps output; eps_max input; omg_max input; p_init local; fi_r local; t_r local; t_tek local; t1 local; t2 local; t3 local; fi input; traz output; priz_raz input
